simulink model "two_virtual_wheel_subsystems"  (R2018a)
settings: Solver=ode3  StartTime=0.0  StopTime=tfinal  FixedStep=.002  RelTol=1e-3  EnableMultiTasking=on
InitFcn:
  | two_virtual_wheel_params
values from neighbouring files (symbols this model uses):
  b1 = T1*k1    (= 0.15)    [two_virtual_wheel_params.m]    (also in two_virtual_wheels.m)
  b2 = T2*k2    (= 0.015)    [two_virtual_wheel_params.m]    (also in two_virtual_wheels.m)
  Jw1 = .5*1.5/4    (= 0.1875)    [two_virtual_wheel_params.m]    (also in two_virtual_wheels.m)
  Jw2 = .5*.015/4    (= 0.001875)    [two_virtual_wheel_params.m]    (also in two_virtual_wheels.m = 0.146)
  k1 = .5*15    (= 7.5)    [two_virtual_wheel_params.m]    (also in two_virtual_wheels.m)
  k2 = .5*15    (= 7.5)    [two_virtual_wheel_params.m]    (also in two_virtual_wheels.m)
  step_time = 1    [two_virtual_wheel_params.m]    (also in two_virtual_wheels.m)
  T2 = 1/500    (= 0.002)    [two_virtual_wheel_params.m]    (also in two_virtual_wheels.m)
  Theta_z_0 = 45    [two_virtual_wheel_params.m]    (also in two_virtual_wheels.m)
undefined symbols (not defined in the file or in its folder): DiscIntNeverNeededParam
libraries: simulink x2
settings Model: ExtModeTrigMode=oneshot  ExtModeArmWhenConnect=off  Creator=jfr  LastModifiedBy=salman
settings DataIOCC: SaveFormat=Array  SignalLoggingSaveFormat=ModelDataLogs  TimeSaveName=tout2  OutputSaveName=yout2  SignalLoggingName=sigsOut
settings OptimizationCC: BooleanDataType=off  ExpressionDepthLimit=2147483647  InitFltsAndDblsToZero=on  LifeSpan=inf
settings DebuggingCC: SaveWithParameterizedLinksMsg=none  UnderspecifiedInitializationDetection=Classic  MergeDetectMultiDrivingBlocksExec=none  SignalResolutionControl=TryResolveAllWithWarning  MultiTaskDSMMsg=warning  MultiTaskCondExecSysMsg=none  FcnCallInpInsideContextMsg=warning  AllowSymbolicDim=off  StateNameClashWarn=warning  SFUnexpectedBacktrackingDiag=warning  SFNoUnconditionalDefaultTransitionDiag=warning  SFExecutionAtInitializationDiag=none
settings HardwareCC: ProdBitPerPointer=32  ProdBitPerSizeT=32  ProdBitPerPtrDiffT=32  ProdLargestAtomicFloat=None  ProdIntDivRoundTo=Undefined  ProdEndianess=Unspecified  ProdWordSize=32  ProdHWDeviceType=32-bit Generic  TargetUnknown=on
settings ModelReferenceCC: PropagateSignalLabelsOutOfModel=off
settings CodeAppCC: StateflowObjectComments=on
settings GRTTargetCC: TargetFcnLib=ansi_tfl_tmw.mat  TargetLangStandard=C89/C90 (ANSI)  GeneratePreprocessorConditionals=Disable all  CombineOutputUpdateFcns=off  GRTInterface=on
settings ConfigComp: CovMetricSettings=dw  CovHtmlReporting=on  CovSaveCumulativeToWorkspaceVar=on  CovSaveSingleToWorkspaceVar=on  CovExternalEMLEnable=off

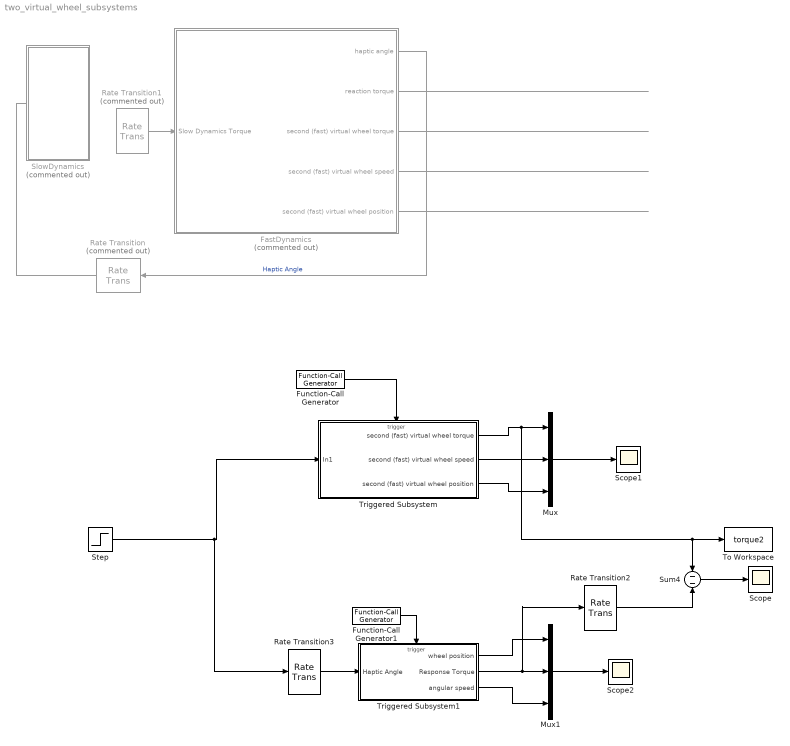
== system two_virtual_wheel_subsystems ==
  FastDynamics : Subsystem  Commented=on
  Function-Call Generator : simulink/Ports & Subsystems/Function-Call Generator  sample_time=0.002  numberOfIterations=1
  Function-Call Generator1 : simulink/Ports & Subsystems/Function-Call Generator  sample_time=0.02  numberOfIterations=1
  Mux : Mux  Inputs=3
  Mux1 : Mux  Inputs=3
  Rate Transition : RateTransition  Commented=on
  Rate Transition1 : RateTransition  Commented=on
  Rate Transition2 : RateTransition
  Rate Transition3 : RateTransition
  Scope : Scope
  Scope1 : Scope
  Scope2 : Scope
  SlowDynamics : Subsystem  Commented=on
  Step : Step  Time=step_time  After=Theta_z_0  SampleTime=0
  Sum4 : Sum  Inputs=-|-  SaturateOnIntegerOverflow=on  InputSameDT=on  OutDataTypeStr=Inherit: Same as first input
  To Workspace : ToWorkspace  VariableName=torque2  SampleTime=-1
  Triggered Subsystem : Subsystem  TreatAsAtomicUnit=on
  Triggered Subsystem1 : Subsystem  TreatAsAtomicUnit=on
  wires:
  FastDynamics/2(reaction torque) -> ?
  FastDynamics/3(second (fast) virtual wheel torque) -> ?
  FastDynamics/4(second (fast) virtual wheel speed) -> ?
  FastDynamics/5(second (fast) virtual wheel position) -> ?
  FastDynamics/1(haptic angle) -> Rate Transition/1  "Haptic Angle"
  ? -> ?
  ? -> Rate Transition1/1
  Rate Transition1/1 -> FastDynamics/1(Slow Dynamics Torque)
  Rate Transition/1 -> ?
  Sum4/1 -> Scope/1
  Function-Call Generator/1 -> Triggered Subsystem/Trigger
  Triggered Subsystem/1(second (fast) virtual wheel torque) -> To Workspace/1, Sum4/1, Mux/1
  Triggered Subsystem/2(second (fast) virtual wheel speed) -> Mux/2
  Triggered Subsystem/3(second (fast) virtual wheel position) -> Mux/3
  Triggered Subsystem1/2(Response Torque) -> Rate Transition2/1, Mux1/2
  Triggered Subsystem1/1(wheel position) -> Mux1/1
  Triggered Subsystem1/3(angular speed) -> Mux1/3
  Mux/1 -> Scope1/1
  Mux1/1 -> Scope2/1
  Rate Transition2/1 -> Sum4/2
  Function-Call Generator1/1 -> Triggered Subsystem1/Trigger
  Rate Transition3/1 -> Triggered Subsystem1/1(Haptic Angle)
  Step/1 -> Rate Transition3/1, Triggered Subsystem/1(In1)

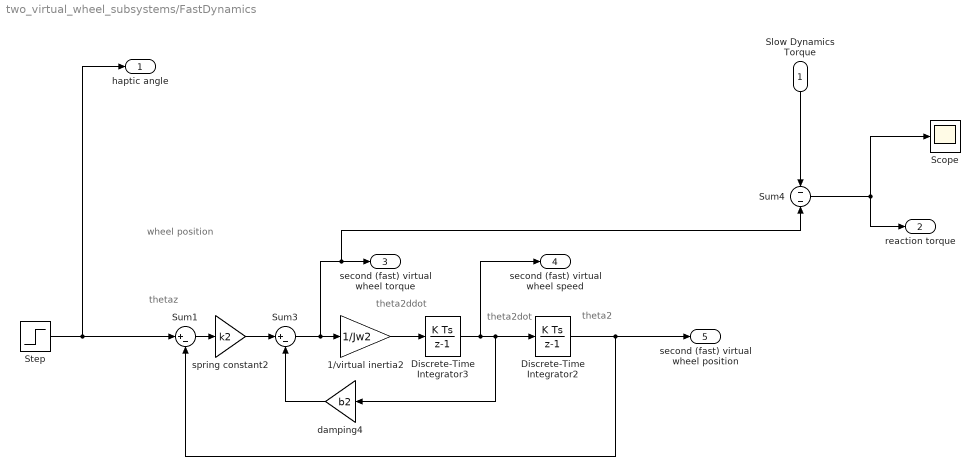
== system two_virtual_wheel_subsystems/FastDynamics ==
  note: theta2
  note: theta2dot
  note: theta2ddot
  note: thetaz
  note: wheel position
  Slow Dynamics Torque : Inport
  1/virtual inertia2 : Gain  Gain=1/Jw2  SaturateOnIntegerOverflow=on  OutDataTypeStr=Inherit: Same as input  ParamDataTypeStr=Inherit: Same as input
  Discrete-Time Integrator2 : DiscreteIntegrator  SampleTime=-1  ICPrevOutput=DiscIntNeverNeededParam  ICPrevScaledInput=DiscIntNeverNeededParam
  Discrete-Time Integrator3 : DiscreteIntegrator  SampleTime=-1  ICPrevOutput=DiscIntNeverNeededParam  ICPrevScaledInput=DiscIntNeverNeededParam
  Scope : Scope
  Step : Step  Time=step_time  After=Theta_z_0  SampleTime=T2
  Sum1 : Sum  Inputs=|+-  SaturateOnIntegerOverflow=on  InputSameDT=on  OutDataTypeStr=Inherit: Same as first input
  Sum3 : Sum  Inputs=|+-  SaturateOnIntegerOverflow=on  InputSameDT=on  OutDataTypeStr=Inherit: Same as first input
  Sum4 : Sum  Inputs=-|-  SaturateOnIntegerOverflow=on  InputSameDT=on  OutDataTypeStr=Inherit: Same as first input
  damping4 : Gain  Gain=b2  SaturateOnIntegerOverflow=on  OutDataTypeStr=Inherit: Same as input  ParamDataTypeStr=Inherit: Same as input
  spring constant2 : Gain  Gain=k2  SaturateOnIntegerOverflow=on  OutDataTypeStr=Inherit: Same as input  ParamDataTypeStr=Inherit: Same as input
  haptic angle : Outport
  reaction torque : Outport  Port=2
  second (fast) virtual wheel torque : Outport  Port=3
  second (fast) virtual wheel speed : Outport  Port=4
  second (fast) virtual wheel position : Outport  Port=5
  wires:
  spring constant2/1 -> Sum3/1
  damping4/1 -> Sum3/2
  1/virtual inertia2/1 -> Discrete-Time Integrator3/1
  Discrete-Time Integrator2/1 -> second (fast) virtual wheel position/1, Sum1/2
  Sum4/1 -> reaction torque/1, Scope/1
  Slow Dynamics Torque/1 -> Sum4/1
  Sum1/1 -> spring constant2/1
  Step/1 -> haptic angle/1, Sum1/1
  Discrete-Time Integrator3/1 -> second (fast) virtual wheel speed/1, Discrete-Time Integrator2/1, damping4/1
  Sum3/1 -> 1/virtual inertia2/1, second (fast) virtual wheel torque/1, Sum4/2

== system two_virtual_wheel_subsystems/SlowDynamics ==

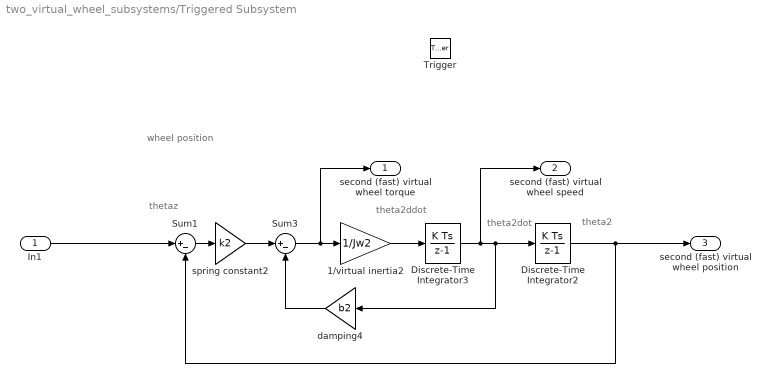
== system two_virtual_wheel_subsystems/Triggered Subsystem ==
  note: theta2
  note: theta2dot
  note: thetaz
  note: wheel position
  note: theta2ddot
  In1 : Inport
  Trigger : TriggerPort  TriggerType=function-call  VariantControl=Variant
  1/virtual inertia2 : Gain  Gain=1/Jw2  SaturateOnIntegerOverflow=on  OutDataTypeStr=Inherit: Same as input  ParamDataTypeStr=Inherit: Same as input
  Discrete-Time Integrator2 : DiscreteIntegrator  SampleTime=-1  ICPrevOutput=DiscIntNeverNeededParam  ICPrevScaledInput=DiscIntNeverNeededParam
  Discrete-Time Integrator3 : DiscreteIntegrator  SampleTime=-1  ICPrevOutput=DiscIntNeverNeededParam  ICPrevScaledInput=DiscIntNeverNeededParam
  Sum1 : Sum  Inputs=|+-  SaturateOnIntegerOverflow=on  InputSameDT=on  OutDataTypeStr=Inherit: Same as first input
  Sum3 : Sum  Inputs=|+-  SaturateOnIntegerOverflow=on  InputSameDT=on  OutDataTypeStr=Inherit: Same as first input
  damping4 : Gain  Gain=b2  SaturateOnIntegerOverflow=on  OutDataTypeStr=Inherit: Same as input  ParamDataTypeStr=Inherit: Same as input
  spring constant2 : Gain  Gain=k2  SaturateOnIntegerOverflow=on  OutDataTypeStr=Inherit: Same as input  ParamDataTypeStr=Inherit: Same as input
  second (fast) virtual wheel torque : Outport
  second (fast) virtual wheel speed : Outport  Port=2
  second (fast) virtual wheel position : Outport  Port=3
  wires:
  Discrete-Time Integrator2/1 -> second (fast) virtual wheel position/1, Sum1/2
  damping4/1 -> Sum3/2
  Discrete-Time Integrator3/1 -> second (fast) virtual wheel speed/1, Discrete-Time Integrator2/1, damping4/1
  1/virtual inertia2/1 -> Discrete-Time Integrator3/1
  Sum1/1 -> spring constant2/1
  In1/1 -> Sum1/1
  spring constant2/1 -> Sum3/1
  Sum3/1 -> 1/virtual inertia2/1, second (fast) virtual wheel torque/1

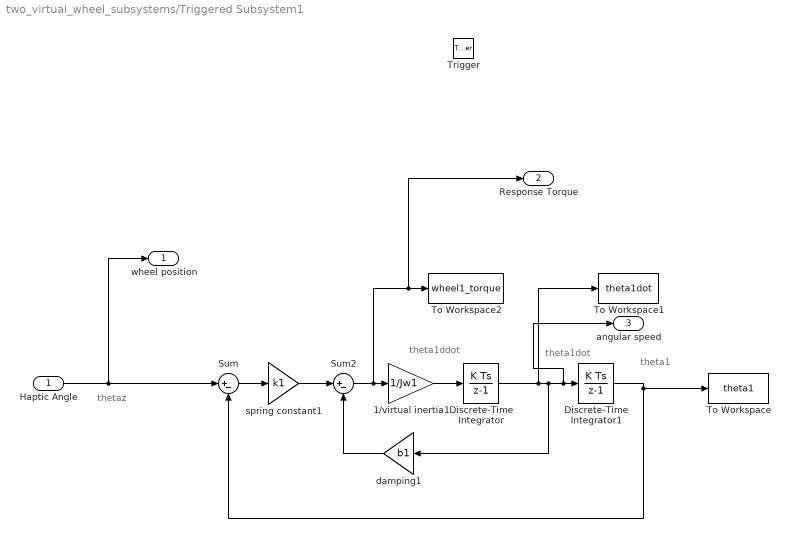
== system two_virtual_wheel_subsystems/Triggered Subsystem1 ==
  note: theta1
  note: theta1dot
  note: theta1ddot
  note: thetaz
  Haptic Angle : Inport
  Trigger : TriggerPort  TriggerType=function-call  VariantControl=Variant
  1/virtual inertia1 : Gain  Gain=1/Jw1  SaturateOnIntegerOverflow=on  OutDataTypeStr=Inherit: Same as input  ParamDataTypeStr=Inherit: Same as input
  Discrete-Time Integrator : DiscreteIntegrator  SampleTime=-1  ICPrevOutput=DiscIntNeverNeededParam  ICPrevScaledInput=DiscIntNeverNeededParam
  Discrete-Time Integrator1 : DiscreteIntegrator  SampleTime=-1  ICPrevOutput=DiscIntNeverNeededParam  ICPrevScaledInput=DiscIntNeverNeededParam
  Sum : Sum  Inputs=|+-  SaturateOnIntegerOverflow=on  InputSameDT=on  OutDataTypeStr=Inherit: Same as first input
  Sum2 : Sum  Inputs=|+-  SaturateOnIntegerOverflow=on  InputSameDT=on  OutDataTypeStr=Inherit: Same as first input
  To Workspace : ToWorkspace  VariableName=theta1  SaveFormat=Structure With Time  SampleTime=-1
  To Workspace1 : ToWorkspace  VariableName=theta1dot  SaveFormat=Structure With Time  SampleTime=-1
  To Workspace2 : ToWorkspace  VariableName=wheel1_torque  SaveFormat=Structure With Time  SampleTime=-1
  damping1 : Gain  Gain=b1  SaturateOnIntegerOverflow=on  OutDataTypeStr=Inherit: Same as input  ParamDataTypeStr=Inherit: Same as input
  spring constant1 : Gain  Gain=k1  SaturateOnIntegerOverflow=on  OutDataTypeStr=Inherit: Same as input  ParamDataTypeStr=Inherit: Same as input
  wheel position : Outport
  Response Torque : Outport  Port=2
  angular speed : Outport  Port=3
  wires:
  spring constant1/1 -> Sum2/1
  Sum/1 -> spring constant1/1
  1/virtual inertia1/1 -> Discrete-Time Integrator/1
  Discrete-Time Integrator1/1 -> Sum/2, To Workspace/1
  damping1/1 -> Sum2/2
  Haptic Angle/1 -> Sum/1, wheel position/1
  Discrete-Time Integrator/1 -> angular speed/1, Discrete-Time Integrator1/1, damping1/1, To Workspace1/1
  Sum2/1 -> 1/virtual inertia1/1, Response Torque/1, To Workspace2/1
